simulink model "jlty08022311"  (R2022b)
settings: Solver=VariableStepAuto  StartTime=0.0  StopTime=0.2  RelTol=1e-3
libraries: spsVoltageMeasurementLib x7, spsThyristorLib x6, spsACVoltageSourceLib x3, spsGroundLib x1, powerlib_extras x1, spsThreePhaseSeriesRLCBranchLib x1, spsThreePhaseVIMeasurementLib x1, sps_lib x1
settings Model: Creator=赵晨琨  LastModifiedBy=ASUS
settings SolverCC: AlgebraicLoopSolver=TrustRegion
settings DataIOCC: Refine=3
settings DebuggingCC: UnconnectedInputMsg=warning  UnconnectedOutputMsg=warning  UnconnectedLineMsg=warning  SFMachineParentedDataDiag=warning
settings ModelReferenceCC: EnableRefExpFcnMdlSchedulingChecks=on

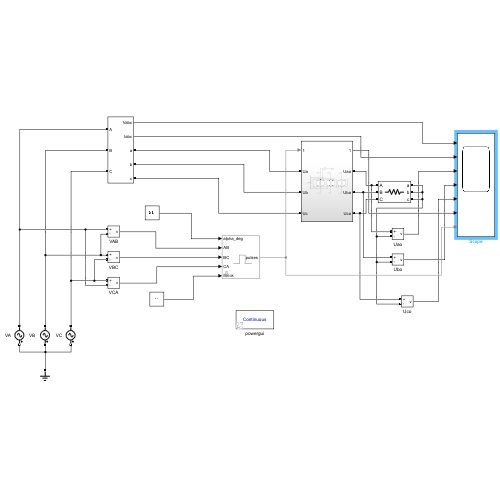
[thumbnail: Simulink's stored preview of the top-level diagram]
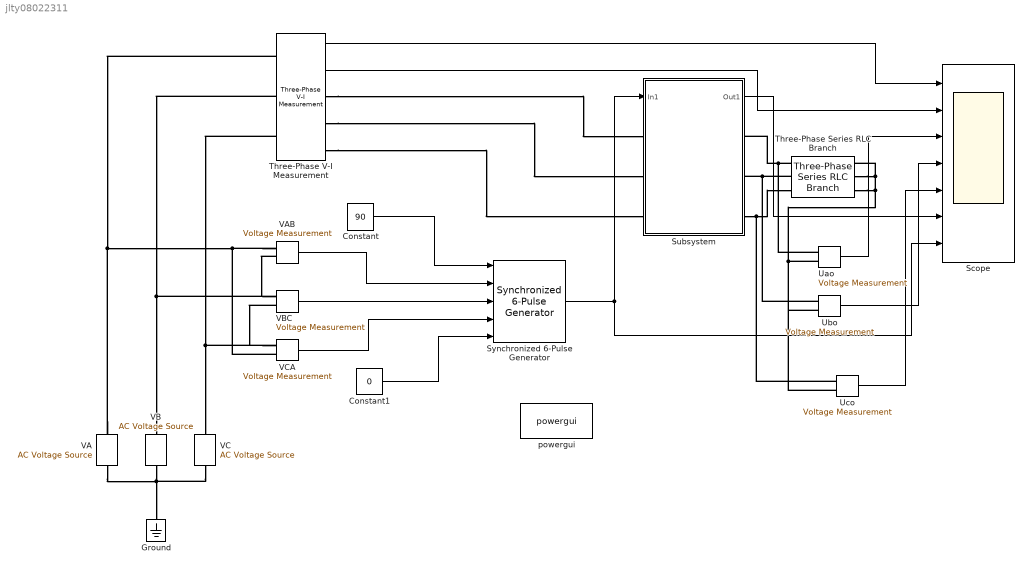
== system jlty08022311 ==
  Constant : Constant  Value=90  VectorParams1D=off
  Constant1 : Constant  Value=0
  Ground : spsGroundLib/Ground  LConnTagsString=a
  Scope : Scope  NumInputPorts=7
  Subsystem : Subsystem
  Synchronized 6-Pulse Generator : powerlib_extras/Control  Blocks/Synchronized 6-Pulse Generator  freq=50  pwidth=10  Double_Pulse=on
  Three-Phase Series RLC Branch : spsThreePhaseSeriesRLCBranchLib/Three-Phase Series RLC Branch  LConnTagsString=A|B|C  RConnTagsString=A|B|C  BranchType=R  Resistance=1  Inductance=1e-3  Capacitance=1e-6  Measurements=None
  Three-Phase V-I Measurement : spsThreePhaseVIMeasurementLib/Three-Phase V-I Measurement  VoltageMeasurement=phase-to-ground  SetLabelV=off  LabelV=Vabc  Vpu=off  VpuLL=off  CurrentMeasurement=yes  SetLabelI=off  LabelI=Iabc  Ipu=off  Pbase=100e6  Vbase=500e3  OutputType=Complex  PhasorSimulation=off  PSBequivalent=0
  Uao : spsVoltageMeasurementLib/Voltage Measurement  PhasorSimulation=off  OutputType=Complex  PSBequivalent=0
  Ubo : spsVoltageMeasurementLib/Voltage Measurement  PhasorSimulation=off  OutputType=Complex  PSBequivalent=0
  Uco : spsVoltageMeasurementLib/Voltage Measurement  PhasorSimulation=off  OutputType=Complex  PSBequivalent=0
  VA : spsACVoltageSourceLib/AC Voltage Source  Amplitude=311  Phase=0  Frequency=50  SampleTime=0  Measurements=None  BusType=swing  Pref=10e3  Qref=0  Qmin=-inf  Qmax=+inf
  VAB : spsVoltageMeasurementLib/Voltage Measurement  PhasorSimulation=off  OutputType=Complex  PSBequivalent=0
  "VB " : spsACVoltageSourceLib/AC Voltage Source  Amplitude=311  Phase=-120  Frequency=50  SampleTime=0  Measurements=None  BusType=swing  Pref=10e3  Qref=0  Qmin=-inf  Qmax=+inf
  VBC : spsVoltageMeasurementLib/Voltage Measurement  PhasorSimulation=off  OutputType=Complex  PSBequivalent=0
  VC : spsACVoltageSourceLib/AC Voltage Source  Amplitude=311  Phase=120  Frequency=50  SampleTime=0  Measurements=None  BusType=swing  Pref=10e3  Qref=0  Qmin=-inf  Qmax=+inf
  VCA : spsVoltageMeasurementLib/Voltage Measurement  PhasorSimulation=off  OutputType=Complex  PSBequivalent=0
  powergui : sps_lib/powergui  Priority=1  SimulationMode=Continuous  SampleTime=5e-5  frequency=60  Iterations=50  frequencyindice=50  Pbase=100e6  ErrMax=1e-4  UnitsV=kV  UnitsW=MW  buscounter=0  FunctionMessages=off  echomessages=off  EnableUseOfTLC=off  CurrentSourceSwitches=off  DisableSnubberDevices=off  DisableRonSwitches=off  DisableVfSwitches=off  DisplayEquations=off  AutomaticDiscreteSolvers=off  SolverType=Tustin/Backward Euler (TBE)  Interpol=off  ExternalGateDelay=off  methode=off  Ts=100  x0status=blocks  SPID=on  SwTol=0  HookPort=off  NonlinearTolerance=1e-4  nMaxIteration=100  ContinueOnMaxIteration=off  RestoreLinks=warning  ResistiveCurrentMeasurement=off  Frange=[0:2:500]  Ylog=off  Xlog=on  ShowGrid=off  save=off  variable=ZData  structure=0  ZoomFFT=off  StartTime=0.0  cycles=1  DisplayStyle=1  fundamental=60  FreqAxis=off  MaxFrequency=1000  frequencyindicesteady=1  RmsSteady=1  display=off
  wires:
  Constant1/1 -> Synchronized 6-Pulse Generator/5
  Constant/1 -> Synchronized 6-Pulse Generator/1
  VAB/1 -> Synchronized 6-Pulse Generator/2
  VBC/1 -> Synchronized 6-Pulse Generator/3
  VCA/1 -> Synchronized 6-Pulse Generator/4
  Three-Phase V-I Measurement/1 -> Scope/1
  Three-Phase V-I Measurement/2 -> Scope/2
  Synchronized 6-Pulse Generator/1 -> Subsystem/1(In1), Scope/7
  Uao/1 -> Scope/3
  Ubo/1 -> Scope/4
  Uco/1 -> Scope/5
  Subsystem/1(Out1) -> Scope/6
  connections:
  VA/RConn1 -- VC/RConn1 -- "VB "/RConn1 -- Ground/LConn1
  VA/LConn1 -- VAB/LConn1 -- VCA/LConn2 -- Three-Phase V-I Measurement/LConn1
  VAB/LConn2 -- VBC/LConn1 -- Three-Phase V-I Measurement/LConn2 -- "VB "/LConn1
  VCA/LConn1 -- VBC/LConn2 -- Three-Phase V-I Measurement/LConn3 -- VC/LConn1
  Three-Phase V-I Measurement/RConn1 -- Subsystem/LConn1
  Three-Phase V-I Measurement/RConn2 -- Subsystem/LConn2
  Three-Phase V-I Measurement/RConn3 -- Subsystem/LConn3
  Three-Phase Series RLC Branch/LConn2 -- Ubo/LConn1 -- Subsystem/RConn2
  Three-Phase Series RLC Branch/LConn1 -- Uao/LConn1 -- Subsystem/RConn1
  Subsystem/RConn3 -- Uco/LConn1 -- Three-Phase Series RLC Branch/LConn3
  Uao/LConn2 -- Uco/LConn2 -- Ubo/LConn2 -- Three-Phase Series RLC Branch/RConn3 -- Three-Phase Series RLC Branch/RConn2 -- Three-Phase Series RLC Branch/RConn1

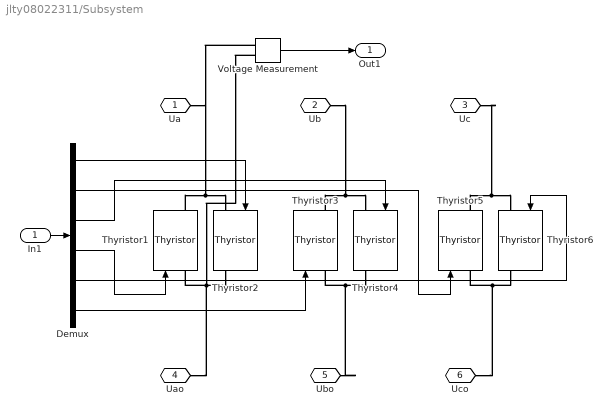
== system jlty08022311/Subsystem ==
  In1 : Inport
  Demux : Demux  Outputs=6
  Thyristor{1..6} (6 alike) : spsThyristorLib/Thyristor  Ron=0.00001  Lon=0  Vf=0.8  IC=0  Rs=500  Cs=250e-9  Measurements=on
  Voltage Measurement : spsVoltageMeasurementLib/Voltage Measurement  PhasorSimulation=off  OutputType=Complex  PSBequivalent=0
  Ua : PMIOPort  Side=Left
  Ub : PMIOPort  Port=2  Side=Left
  Uc : PMIOPort  Port=3  Side=Left
  Uao : PMIOPort  Port=4  Side=Right
  Ubo : PMIOPort  Port=5  Side=Right
  Uco : PMIOPort  Port=6  Side=Right
  Out1 : Outport
  wires:
  In1/1 -> Demux/1
  Demux/1 -> Thyristor2/1
  Demux/4 -> Thyristor1/1
  Demux/2 -> Thyristor5/1
  Demux/5 -> Thyristor6/1
  Demux/3 -> Thyristor4/1
  Demux/6 -> Thyristor3/1
  Voltage Measurement/1 -> Out1/1
  connections:
  Thyristor1/RConn1 -- Voltage Measurement/LConn1 -- Ua/RConn1 -- Thyristor2/LConn1
  Thyristor2/RConn1 -- Voltage Measurement/LConn2 -- Uao/RConn1 -- Thyristor1/LConn1
  Thyristor3/RConn1 -- Ub/RConn1 -- Thyristor4/LConn1
  Thyristor4/RConn1 -- Ubo/RConn1 -- Thyristor3/LConn1
  Thyristor5/RConn1 -- Uc/RConn1 -- Thyristor6/LConn1
  Thyristor6/RConn1 -- Uco/RConn1 -- Thyristor5/LConn1
